simulink model "gm_sampleModel1956_1_sub"  (R2023a)
settings: Solver=VariableStepAuto  StartTime=0.0  StopTime=10.0  RelTol=1e-3
libraries: simulink x3
settings Model: Creator=user1  LastModifiedBy=user1
settings OptimizationCC: BlockReduction=off  ConditionallyExecuteInputs=off
settings DebuggingCC: InheritedTsInSrcMsg=none

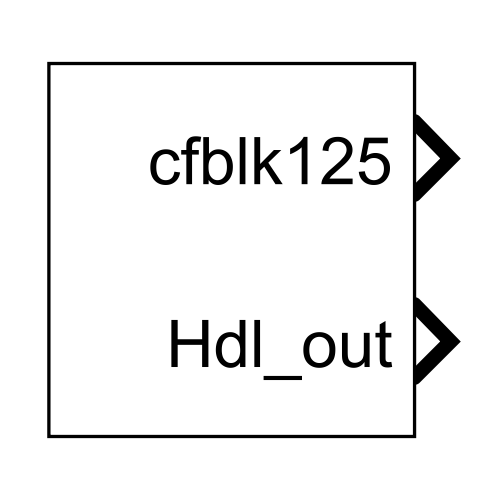
[thumbnail: Simulink's stored preview of the top-level diagram]
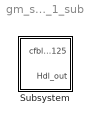
== system gm_sampleModel1956_1_sub ==
  Subsystem : Subsystem

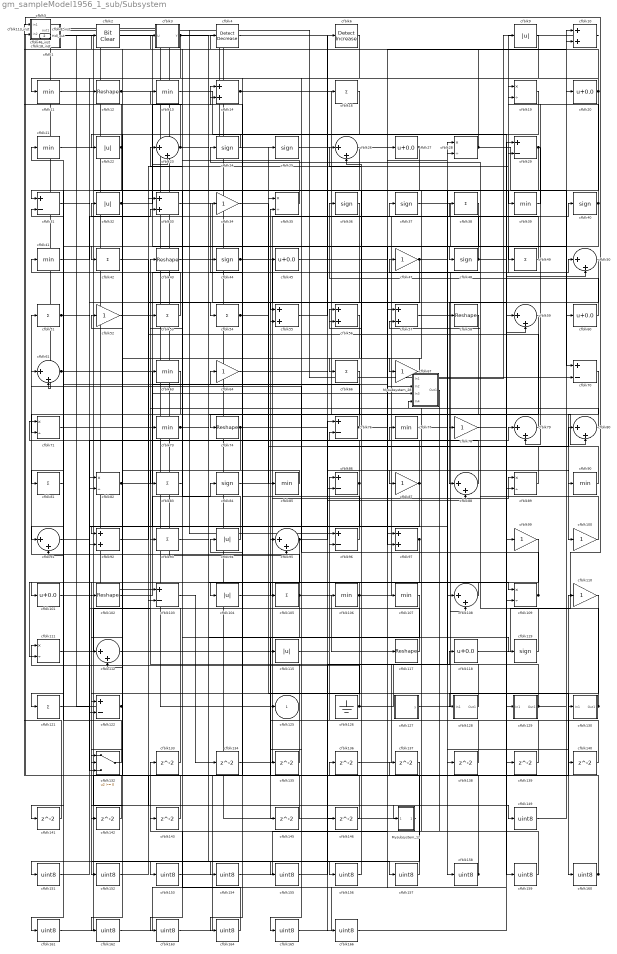
== system gm_sampleModel1956_1_sub/Subsystem ==
  Mysubsystem_12 : Subsystem
  Mysubsystem_28 : Subsystem
  cfblk1 : Subsystem  mask(Compare To Zero){relop=<=, OutDataTypeStr=uint8, ZeroCross=on}
      mask prompts: relop "Simulink:masks:Operator_MP"; OutDataTypeStr "Simulink:masks:OutputDataType_MP"; ZeroCross "Simulink:masks:EnableZerocrossingDetection_MP"
      mask help: Simulink:masks:CompareToZero_MD
      mask init:
      | OutDataTypeStr = 'uint8';
      | ZeroCross = 'on';
      | blkName = 'sampleModel1956_1_sub/Subsystem/cfblk1';
      | relop = '<=';
      | setValue = 'fixdt(0, 8)';
      mask TypeOptions relop: == | ~= | < | <= | >= | >
      mask TypeOptions OutDataTypeStr: Simulink:masks:uint8 | Simulink:masks:boolean
      mask Callback ZeroCross: sl('zeroCrossEnable', gcbh);
      mask Display: disp([relop,' 0'])
  cfblk{10,14,33,55..57,92,97} (8 alike) : Sum  OutDataTypeStr=uint8
  cfblk{34,47,52,64,67,78,87,99..100,110} (10 alike) : Gain  OutDataTypeStr=uint8
  cfblk{20,27,45,60,101,118} (6 alike) : Bias  Bias=0.0  SaturateOnIntegerOverflow=off
  cfblk{12,43,58,74,102,117} (6 alike) : Reshape
  cfblk{29,31,70,76,86,96,103,122} (8 alike) : Sum  Inputs=+-  OutDataTypeStr=uint8
  cfblk{9,22,32,94,104,115} (6 alike) : Abs  OutDataTypeStr=uint8  SaturateOnIntegerOverflow=off
  cfblk{16,38,42,49,51,53..54,66,81,83,93,105,121} (13 alike) : Sum  Inputs=+  OutDataTypeStr=uint8
  cfblk{11,13,21,39,41,63,73,77,85,90,106..107} (12 alike) : MinMax  OutDataTypeStr=uint8
  cfblk{23,26,50,59,61,79..80,88,91,95,108,112} (12 alike) : Sum  Inputs=|++  OutDataTypeStr=uint8
  cfblk{19,28,35,71,82,89,109,111} (8 alike) : Product  Inputs=*/  OutDataTypeStr=uint8  RndMeth=Zero  SaturateOnIntegerOverflow=on
  cfblk113_inst : Subsystem
  cfblk{24..25,36..37,40,44,48,84,119} (9 alike) : Signum
  cfblk126 : Ground
  cfblk127 : Subsystem  mask(Counter Free-Running){NumBits=double(16), tsamp=double(-1)}
      mask prompts: NumBits "Simulink:masks:NumberOfBits_MP"; tsamp "Simulink:masks:SampleTime_MP"
      mask help: Simulink:masks:CounterFreeRunning_MD
  cfblk128 : Subsystem
  cfblk129 : Subsystem
  cfblk130 : Subsystem
  cfblk132 : Switch  OutDataTypeStr=uint8  SaturateOnIntegerOverflow=off  InputSameDT=off
  cfblk{133..143,145..146} (13 alike) : Delay  SampleTime=1
  cfblk{149,151..166} (17 alike) : DataTypeConversion  OutDataTypeStr=uint8  SaturateOnIntegerOverflow=off  RndMeth=Floor
  cfblk18_inst : Subsystem
  cfblk2 : simulink/Logic and Bit Operations/Bit Clear  iBit=0
      settings: LibrarySourceBlock=|
      | hdlsllib/Logic and Bit
      | Operations/Bit Clear
  cfblk3 : Subsystem  mask(Detect Rise Positive){vinit=double(0), InputProcessing=Elements as channels (sample based), OutDataTypeStr=uint8}
      mask prompts: vinit "Simulink:masks:InitialCondition_MP"; InputProcessing "Simulink:masks:InputProcessing_MP"; OutDataTypeStr "Simulink:masks:OutputDataType_MP"
      mask help: Simulink:masks:DetectRisePositive_MD
      mask init:
      | InputProcessing = 'Elements as channels (sample based)';
      | OutDataTypeStr = 'uint8';
      | vinit = double(0);
      mask TypeOptions InputProcessing: Simulink:masks:ColumnsAsChannelsFrameBased | Simulink:masks:ElementsAsChannelsSampleBased
      mask TypeOptions OutDataTypeStr: Simulink:masks:uint8 | Simulink:masks:boolean
      mask Display: fprintf('U > 0\n&  NOT\nU/z > 0')
  cfblk4 : simulink/Logic and Bit Operations/Detect Decrease  vinit=0.0  OutDataTypeStr=uint8
      settings: LibrarySourceBlock=|
      | hdlsllib/Logic and Bit
      | Operations/Detect
      | Decrease
  cfblk46_inst : Subsystem
  cfblk5 : Constant  Value=0  OutDataTypeStr=uint8  SampleTime=1
  cfblk6 : simulink/Logic and Bit Operations/Detect Increase  vinit=0.0  OutDataTypeStr=uint8
      settings: LibrarySourceBlock=|
      | hdlsllib/Logic and Bit
      | Operations/Detect
      | Increase
  cfblk8_inst : Subsystem
  cfblk125 : Outport  OutDataTypeStr=uint8  SampleTime=1  VectorParamsAs1DForOutWhenUnconnected=off
  Hdl_out : Outport  Port=2  OutDataTypeStr=uint8  SampleTime=1
  wires:
  Mysubsystem_12/1(Out1) -> cfblk1/1(u)
  Mysubsystem_28/1(Out1) -> cfblk133/1
  cfblk1/1(y) -> cfblk149/1
  cfblk10/1 -> Mysubsystem_28/1(In1)
  cfblk100/1 -> cfblk24/1
  cfblk101/1 -> cfblk156/1
  cfblk102/1 -> cfblk84/1
  cfblk103/1 -> cfblk134/1
  cfblk104/1 -> cfblk109/1
  cfblk105/1 -> cfblk117/1, cfblk145/1, cfblk51/1
  cfblk106/1 -> cfblk40/1, cfblk132/2, cfblk104/1
  cfblk107/1 -> cfblk153/1
  cfblk108/1 -> cfblk102/1
  cfblk109/1 -> cfblk61/1, cfblk26/2
  cfblk11/1 -> cfblk12/1
  cfblk110/1 -> cfblk160/1
  cfblk111/1 -> cfblk43/1
  cfblk112/1 -> cfblk37/1
  cfblk113_inst/1(out1) -> cfblk95/2
  cfblk115/1 -> cfblk86/1
  cfblk117/1 -> cfblk32/1
  cfblk118/1 -> cfblk18_inst/1(in1)
  cfblk119/1 -> cfblk57/2
  cfblk12/1 -> cfblk48/1, cfblk23/2
  cfblk121/1 -> cfblk82/2
  cfblk122/1 -> cfblk52/1, Hdl_out/1
  cfblk126/1 -> cfblk28/2, cfblk111/1
  cfblk127/1(y) -> cfblk9/1
  cfblk128/1(Out1) -> cfblk64/1
  cfblk129/1(Out1) -> cfblk10/2, cfblk93/1
  cfblk13/1 -> cfblk159/1
  cfblk130/1(Out1) -> cfblk47/1, cfblk128/1(In1)
  cfblk132/1 -> cfblk21/1
  cfblk133/1 -> cfblk82/1
  cfblk134/1 -> cfblk89/1
  cfblk135/1 -> cfblk35/2
  cfblk136/1 -> cfblk108/2
  cfblk137/1 -> cfblk151/1
  cfblk138/1 -> cfblk76/2
  cfblk139/1 -> cfblk96/2
  cfblk14/1 -> cfblk139/1, cfblk39/1
  cfblk140/1 -> cfblk55/2
  cfblk141/1 -> cfblk46_inst/1(in1)
  cfblk142/1 -> cfblk8_inst/2(in2)
  cfblk143/1 -> cfblk113_inst/1(in1)
  cfblk145/1 -> cfblk112/2
  cfblk146/1 -> cfblk95/1
  cfblk149/1 -> cfblk20/1
  cfblk151/1 -> cfblk92/2
  cfblk152/1 -> cfblk137/1
  cfblk153/1 -> cfblk29/1
  cfblk154/1 -> cfblk107/1
  cfblk155/1 -> cfblk118/1
  cfblk156/1 -> cfblk56/1
  cfblk157/1 -> cfblk56/2
  cfblk158/1 -> cfblk14/1, cfblk136/1
  cfblk159/1 -> cfblk77/1
  cfblk16/1 -> cfblk112/1
  cfblk160/1 -> cfblk94/1, cfblk26/1
  cfblk161/1 -> cfblk110/1
  cfblk162/1 -> cfblk57/1
  cfblk163/1 -> cfblk99/1
  cfblk164/1 -> cfblk143/1
  cfblk165/1 -> cfblk59/1
  cfblk166/1 -> cfblk59/2
  cfblk18_inst/1(out1) -> cfblk103/1
  cfblk19/1 -> cfblk152/1
  cfblk2/1 -> cfblk85/1
  cfblk20/1 -> cfblk31/1, cfblk113_inst/2(in2), cfblk11/1
  cfblk21/1 -> cfblk108/1
  cfblk22/1 -> cfblk8_inst/1(in1), cfblk101/1
  cfblk23/1 -> cfblk18_inst/2(in2), cfblk119/1
  cfblk24/1 -> cfblk22/1
  cfblk25/1 -> cfblk87/1
  cfblk26/1 -> cfblk42/1
  cfblk27/1 -> cfblk163/1, cfblk161/1, cfblk66/1
  cfblk28/1 -> cfblk60/1, cfblk4/1
  cfblk29/1 -> cfblk79/2, cfblk67/1
  cfblk3/1(Y) -> cfblk80/2, cfblk132/3, cfblk49/1
  cfblk31/1 -> cfblk54/1
  cfblk32/1 -> cfblk14/2, Mysubsystem_28/2(In2)
  cfblk33/1 -> cfblk88/1
  cfblk34/1 -> cfblk130/1(In1)
  cfblk35/1 -> cfblk46_inst/2(in2)
  cfblk36/1 -> cfblk55/1
  cfblk37/1 -> cfblk70/1
  cfblk38/1 -> cfblk81/1
  cfblk39/1 -> cfblk19/1
  cfblk4/1 -> cfblk146/1
  cfblk40/1 -> cfblk122/1, cfblk19/2
  cfblk41/1 -> cfblk33/2
  cfblk42/1 -> Mysubsystem_12/1(In1)
  cfblk43/1 -> cfblk89/2
  cfblk44/1 -> cfblk25/1, cfblk106/1
  cfblk45/1 -> cfblk38/1
  cfblk46_inst/1(out1) -> cfblk96/1, cfblk70/2
  cfblk47/1 -> cfblk97/1, cfblk103/2, cfblk140/1
  cfblk48/1 -> cfblk50/2, cfblk3/1(U)
  cfblk49/1 -> cfblk2/1
  cfblk5/1 -> cfblk61/2, cfblk125/1
  cfblk50/1 -> cfblk78/1
  cfblk51/1 -> cfblk97/2, cfblk91/1
  cfblk52/1 -> cfblk6/1
  cfblk53/1 -> cfblk41/1
  cfblk54/1 -> cfblk50/1, cfblk154/1
  cfblk55/1 -> cfblk16/1
  cfblk56/1 -> cfblk155/1
  cfblk57/1 -> cfblk58/1
  cfblk58/1 -> cfblk86/2
  cfblk59/1 -> cfblk164/1
  cfblk6/1 -> cfblk74/1
  cfblk60/1 -> cfblk36/1
  cfblk61/1 -> cfblk138/1, Mysubsystem_28/3(In3)
  cfblk63/1 -> cfblk91/2
  cfblk64/1 -> cfblk166/1
  cfblk66/1 -> cfblk71/2
  cfblk67/1 -> cfblk132/1
  cfblk70/1 -> cfblk100/1
  cfblk71/1 -> cfblk34/1
  cfblk73/1 -> cfblk109/2, cfblk105/1
  cfblk74/1 -> cfblk92/1, cfblk88/2
  cfblk76/1 -> cfblk31/2, cfblk90/1
  cfblk77/1 -> cfblk158/1
  cfblk78/1 -> cfblk129/1(In1)
  cfblk79/1 -> cfblk33/1
  cfblk8_inst/1(out1) -> cfblk27/1
  cfblk80/1 -> cfblk63/1
  cfblk81/1 -> cfblk121/1
  cfblk82/1 -> cfblk115/1, cfblk10/1, cfblk28/1
  cfblk83/1 -> cfblk23/1
  cfblk84/1 -> cfblk45/1
  cfblk85/1 -> cfblk83/1
  cfblk86/1 -> cfblk135/1, cfblk13/1
  cfblk87/1 -> cfblk122/2, Mysubsystem_28/4(In4), cfblk53/1
  cfblk88/1 -> cfblk71/1
  cfblk89/1 -> cfblk76/1
  cfblk9/1 -> cfblk165/1
  cfblk90/1 -> cfblk35/1
  cfblk91/1 -> cfblk79/1
  cfblk92/1 -> cfblk29/2
  cfblk93/1 -> cfblk157/1
  cfblk94/1 -> cfblk73/1
  cfblk95/1 -> cfblk80/1, cfblk111/2
  cfblk96/1 -> cfblk44/1
  cfblk97/1 -> cfblk142/1, cfblk141/1
  cfblk99/1 -> cfblk162/1

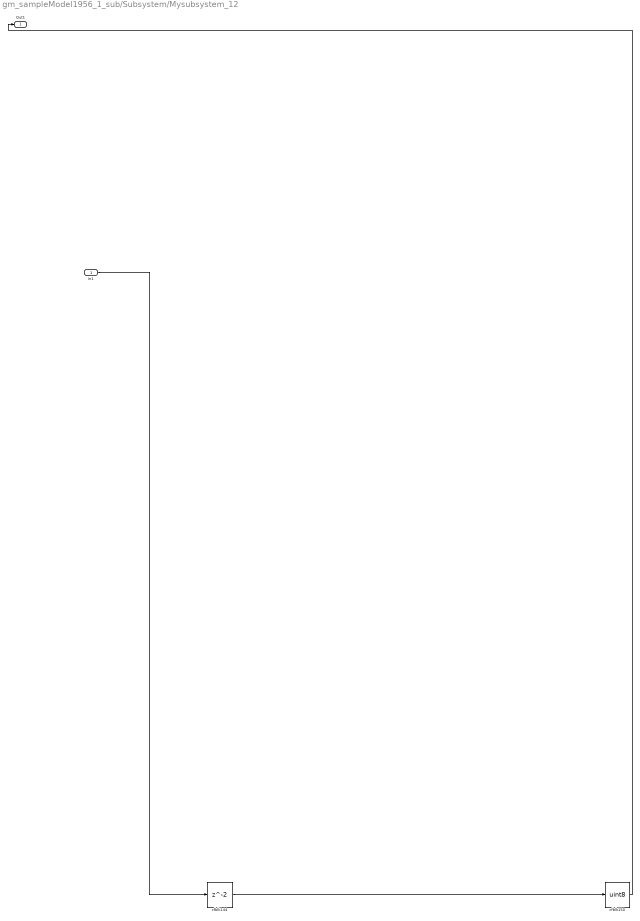
== system gm_sampleModel1956_1_sub/Subsystem/Mysubsystem_12 ==
  In1 : Inport  OutDataTypeStr=uint8  PortDimensions=1  SampleTime=1
  cfblk144 : Delay  SampleTime=1
  cfblk150 : DataTypeConversion  OutDataTypeStr=uint8  SaturateOnIntegerOverflow=off  RndMeth=Floor
  Out1 : Outport  SampleTime=1
  wires:
  In1/1 -> cfblk144/1
  cfblk144/1 -> cfblk150/1
  cfblk150/1 -> Out1/1

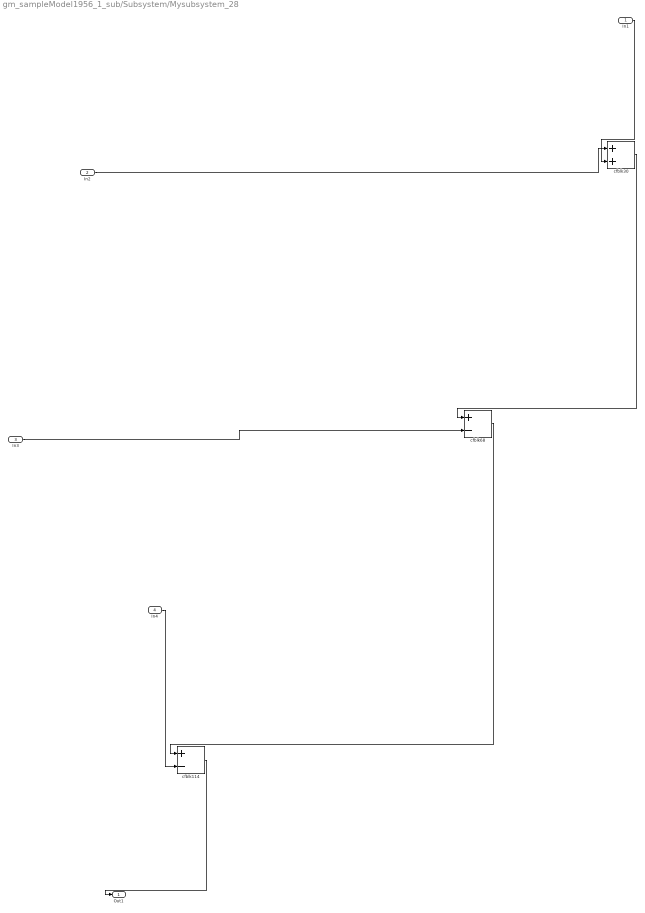
== system gm_sampleModel1956_1_sub/Subsystem/Mysubsystem_28 ==
  In1 : Inport  OutDataTypeStr=uint8  PortDimensions=1  SampleTime=1
  In2 : Inport  Port=2  OutDataTypeStr=uint8  PortDimensions=1  SampleTime=1
  In3 : Inport  Port=3  OutDataTypeStr=uint8  PortDimensions=1  SampleTime=1
  In4 : Inport  Port=4  OutDataTypeStr=uint8  PortDimensions=1  SampleTime=1
  cfblk114 : Sum  Inputs=+-
  cfblk30 : Sum
  cfblk68 : Sum  Inputs=+-
  Out1 : Outport  SampleTime=1
  wires:
  In1/1 -> cfblk30/2
  In2/1 -> cfblk30/1
  In3/1 -> cfblk68/2
  In4/1 -> cfblk114/2
  cfblk114/1 -> Out1/1
  cfblk30/1 -> cfblk68/1
  cfblk68/1 -> cfblk114/1

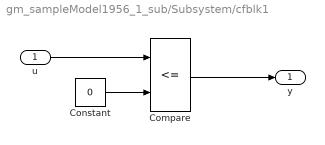
== system gm_sampleModel1956_1_sub/Subsystem/cfblk1 ==
  u : Inport  OutDataTypeStr=uint8  SampleTime=1
  Compare : RelationalOperator  Operator=<=  OutDataTypeStr=fixdt(0, 8)
  Constant : Constant  DisableCoverage=on  Value=0  OutDataTypeStr=Inherit: Inherit via back propagation  SampleTime=-1  PreserveConstantTs=on
  y : Outport  SampleTime=1
  wires:
  u/1 -> Compare/1
  Compare/1 -> y/1
  Constant/1 -> Compare/2

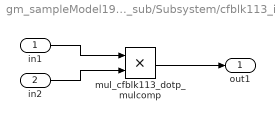
== system gm_sampleModel1956_1_sub/Subsystem/cfblk113_inst ==
  in1 : Inport  OutDataTypeStr=uint8  SampleTime=1
  in2 : Inport  Port=2  OutDataTypeStr=uint8  SampleTime=1
  mul_cfblk113_dotp_mulcomp : Product  Inputs=**  OutDataTypeStr=uint8  SampleTime=1
  out1 : Outport  OutDataTypeStr=uint8  SampleTime=1
  wires:
  in1/1 -> mul_cfblk113_dotp_mulcomp/1
  in2/1 -> mul_cfblk113_dotp_mulcomp/2
  mul_cfblk113_dotp_mulcomp/1 -> out1/1

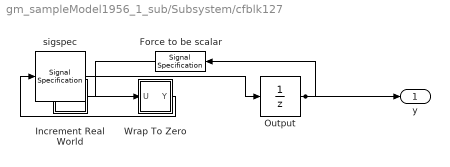
== system gm_sampleModel1956_1_sub/Subsystem/cfblk127 ==
  Force to be scalar : SignalSpecification  DisableCoverage=on  Dimensions=1
  Increment Real World : Subsystem  mask(Real World Value Increment){}
      mask help: Simulink:masks:RealWorldValueIncrement_MD
      mask Display: disp('V++')
  Output : UnitDelay  InitialCondition=0.0  SampleTime=tsamp  HasFrameUpgradeWarning=on
  Wrap To Zero : Subsystem  mask(Wrap To Zero){Threshold=double(65535)}
      mask prompts: Threshold "Simulink:masks:Threshold_MP"
      mask help: Simulink:masks:WrapToZero_MD
  sigspec : SignalSpecification  OutDataTypeStr=uint16  Dimensions=1
  y : Outport  SampleTime=1
  wires:
  Force to be scalar/1 -> Increment Real World/1(u)
  Increment Real World/1(y) -> Wrap To Zero/1(U)
  Output/1 -> Force to be scalar/1, y/1
  Wrap To Zero/1(Y) -> sigspec/1
  sigspec/1 -> Output/1

== system gm_sampleModel1956_1_sub/Subsystem/cfblk128 ==
  In1 : Inport  OutDataTypeStr=uint8  PortDimensions=1  SampleTime=1
  Out1 : Outport  SampleTime=1
  wires:
  In1/1 -> Out1/1

== system gm_sampleModel1956_1_sub/Subsystem/cfblk129 ==
  In1 : Inport  OutDataTypeStr=uint8  PortDimensions=1  SampleTime=1
  Out1 : Outport  SampleTime=1
  wires:
  In1/1 -> Out1/1

== system gm_sampleModel1956_1_sub/Subsystem/cfblk130 ==
  In1 : Inport  OutDataTypeStr=uint8  PortDimensions=1  SampleTime=1
  Out1 : Outport  SampleTime=1
  wires:
  In1/1 -> Out1/1

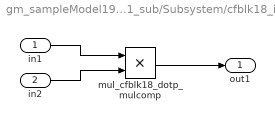
== system gm_sampleModel1956_1_sub/Subsystem/cfblk18_inst ==
  in1 : Inport  OutDataTypeStr=uint8  SampleTime=1
  in2 : Inport  Port=2  OutDataTypeStr=uint8  SampleTime=1
  mul_cfblk18_dotp_mulcomp : Product  Inputs=**  OutDataTypeStr=uint8  SampleTime=1
  out1 : Outport  OutDataTypeStr=uint8  SampleTime=1
  wires:
  in1/1 -> mul_cfblk18_dotp_mulcomp/1
  in2/1 -> mul_cfblk18_dotp_mulcomp/2
  mul_cfblk18_dotp_mulcomp/1 -> out1/1

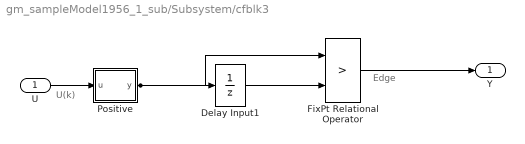
== system gm_sampleModel1956_1_sub/Subsystem/cfblk3 ==
  note: U(k)
  note: Edge
  U : Inport  OutDataTypeStr=uint8  SampleTime=1
  Delay Input1 : UnitDelay  Description=Store in Global RAM  DisableCoverage=on  InitialCondition=vinit  SampleTime=-1  HasFrameUpgradeWarning=on
  FixPt Relational Operator : RelationalOperator  Operator=>  OutDataTypeStr=fixdt(0, 8)  ZeroCross=off  InputSameDT=off
  Positive : Subsystem  mask(Compare To Zero){relop=>, OutDataTypeStr=boolean, ZeroCross=off}
      mask prompts: relop "Simulink:masks:Operator_MP"; OutDataTypeStr "Simulink:masks:OutputDataType_MP"; ZeroCross "Simulink:masks:EnableZerocrossingDetection_MP"
      mask help: Simulink:masks:CompareToZero_MD
      mask init:
      | OutDataTypeStr = 'boolean';
      | ZeroCross = 'off';
      | blkName = 'sampleModel1956_1_sub/Subsystem/cfblk3/Positive';
      | relop = '>';
      | setValue = 'boolean';
      mask TypeOptions relop: == | ~= | < | <= | >= | >
      mask TypeOptions OutDataTypeStr: Simulink:masks:uint8 | Simulink:masks:boolean
      mask Callback ZeroCross: sl('zeroCrossEnable', gcbh);
      mask Display: disp([relop,' 0'])
  Y : Outport  SampleTime=1
  wires:
  U/1 -> Positive/1(u)
  Delay Input1/1 -> FixPt Relational Operator/2
  FixPt Relational Operator/1 -> Y/1
  Positive/1(y) -> FixPt Relational Operator/1, Delay Input1/1

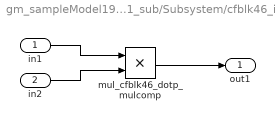
== system gm_sampleModel1956_1_sub/Subsystem/cfblk46_inst ==
  in1 : Inport  OutDataTypeStr=uint8  SampleTime=1
  in2 : Inport  Port=2  OutDataTypeStr=uint8  SampleTime=1
  mul_cfblk46_dotp_mulcomp : Product  Inputs=**  OutDataTypeStr=uint8  SampleTime=1
  out1 : Outport  OutDataTypeStr=uint8  SampleTime=1
  wires:
  in1/1 -> mul_cfblk46_dotp_mulcomp/1
  in2/1 -> mul_cfblk46_dotp_mulcomp/2
  mul_cfblk46_dotp_mulcomp/1 -> out1/1

== system gm_sampleModel1956_1_sub/Subsystem/cfblk8_inst ==
  in1 : Inport  OutDataTypeStr=uint8  SampleTime=1
  in2 : Inport  Port=2  OutDataTypeStr=uint8  SampleTime=1
  mul_cfblk8_dotp_mulcomp : Product  Inputs=**  OutDataTypeStr=uint8  SampleTime=1
  out1 : Outport  OutDataTypeStr=uint8  SampleTime=1
  wires:
  in1/1 -> mul_cfblk8_dotp_mulcomp/1
  in2/1 -> mul_cfblk8_dotp_mulcomp/2
  mul_cfblk8_dotp_mulcomp/1 -> out1/1

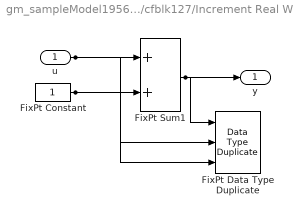
== system gm_sampleModel1956_1_sub/Subsystem/cfblk127/Increment Real World ==
  u : Inport  OutDataTypeStr=uint16  SampleTime=1
  FixPt Constant : Constant  DisableCoverage=on  OutDataTypeStr=Inherit: Inherit via back propagation  SampleTime=-1
  FixPt Data Type Duplicate : DataTypeDuplicate  DisableCoverage=on  NumInputPorts=3
  FixPt Sum1 : Sum  InputSameDT=on  OutDataTypeStr=Inherit: Inherit via back propagation  LockScale=on
  y : Outport  SampleTime=1
  wires:
  u/1 -> FixPt Sum1/1, FixPt Data Type Duplicate/2
  FixPt Constant/1 -> FixPt Sum1/2, FixPt Data Type Duplicate/3
  FixPt Sum1/1 -> FixPt Data Type Duplicate/1, y/1

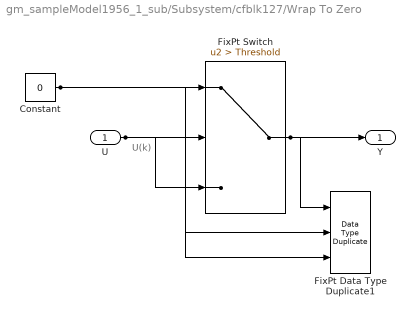
== system gm_sampleModel1956_1_sub/Subsystem/cfblk127/Wrap To Zero ==
  note: U(k)
  U : Inport  OutDataTypeStr=uint16  SampleTime=1
  Constant : Constant  DisableCoverage=on  Value=0  OutDataTypeStr=Inherit: Inherit via back propagation  SampleTime=-1
  FixPt Data Type Duplicate1 : DataTypeDuplicate  DisableCoverage=on  NumInputPorts=3
  FixPt Switch : Switch  Criteria=u2 > Threshold  Threshold=Threshold  OutDataTypeStr=Inherit: Inherit via back propagation  ZeroCross=off  SaturateOnIntegerOverflow=off  InputSameDT=off
  Y : Outport  SampleTime=1
  wires:
  U/1 -> FixPt Switch/3, FixPt Switch/2, FixPt Data Type Duplicate1/2
  Constant/1 -> FixPt Switch/1, FixPt Data Type Duplicate1/3
  FixPt Switch/1 -> FixPt Data Type Duplicate1/1, Y/1

== system gm_sampleModel1956_1_sub/Subsystem/cfblk3/Positive ==
  u : Inport  OutDataTypeStr=uint8  SampleTime=1
  Compare : RelationalOperator  Operator=>  OutDataTypeStr=boolean  ZeroCross=off
  Constant : Constant  DisableCoverage=on  Value=0  OutDataTypeStr=Inherit: Inherit via back propagation  SampleTime=-1  PreserveConstantTs=on
  y : Outport  SampleTime=1
  wires:
  u/1 -> Compare/1
  Compare/1 -> y/1
  Constant/1 -> Compare/2
